simulink model "laba3"  (R2020b)
settings: Solver=VariableStepAuto  StartTime=0.0  StopTime=20  RelTol=1e-3
undefined symbols (not defined in the file): A, b, C, G, L, V, W
libraries: simulink x2
settings Model: Creator=Dimuss  LastModifiedBy=Dimuss
settings DebuggingCC: UnconnectedInputMsg=none  UnconnectedOutputMsg=none  UnconnectedLineMsg=none  SFMachineParentedDataDiag=error
settings ModelReferenceCC: EnableRefExpFcnMdlSchedulingChecks=off

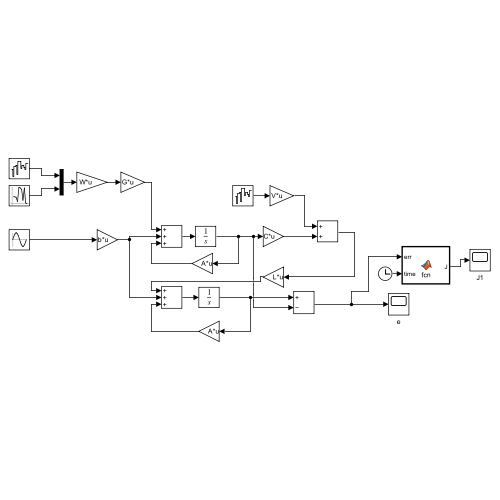
[thumbnail: Simulink's stored preview of the top-level diagram]
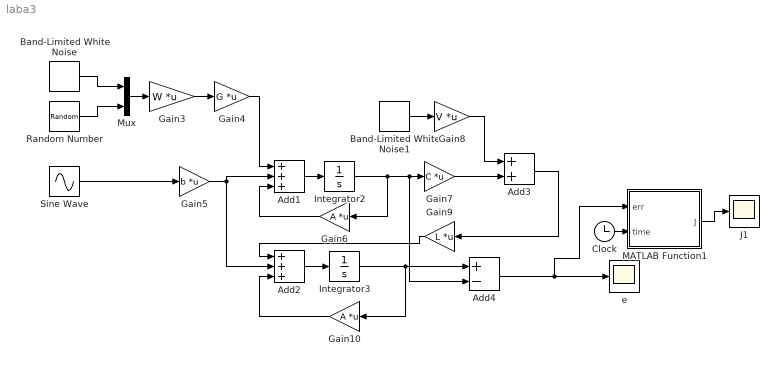
== system laba3 ==
  Add1 : Sum  Inputs=+++
  Add2 : Sum  Inputs=+++
  Add3 : Sum
  Add4 : Sum  Inputs=+-
  Band-Limited White Noise : simulink/Sources/Band-Limited White Noise  Cov=[0.1]  Ts=0.1  seed=[23341]
  Band-Limited White Noise1 : simulink/Sources/Band-Limited White Noise  Cov=[0.1]  Ts=0.1  seed=[23341]
  Clock : Clock
  Gain10 : Gain  Gain=A  Multiplication=Matrix(K*u)
  Gain3 : Gain  Gain=W  Multiplication=Matrix(K*u)
  Gain4 : Gain  Gain=G  Multiplication=Matrix(K*u)
  Gain5 : Gain  Gain=b  Multiplication=Matrix(K*u)
  Gain6 : Gain  Gain=A  Multiplication=Matrix(K*u)
  Gain7 : Gain  Gain=C  Multiplication=Matrix(K*u)
  Gain8 : Gain  Gain=V  Multiplication=Matrix(K*u)
  Gain9 : Gain  Gain=L  Multiplication=Matrix(K*u)
  Integrator2 : Integrator  InitialCondition=[1; 0]
  Integrator3 : Integrator  InitialCondition=[1; 0]
  J1 : Scope
  MATLAB Function1 : MATLAB Function  TreatAsAtomicUnit=on
  Mux : Mux  Inputs=2
  Random Number : RandomNumber  SampleTime=0.1
  Sine Wave : Sin  SampleTime=0
  e : Scope
  wires:
  Band-Limited White Noise/1 -> Mux/1
  Random Number/1 -> Mux/2
  Mux/1 -> Gain3/1
  Gain3/1 -> Gain4/1
  Gain4/1 -> Add1/1
  Gain5/1 -> Add2/2, Add1/2
  Sine Wave/1 -> Gain5/1
  Add1/1 -> Integrator2/1
  Integrator2/1 -> Add4/2, Gain7/1, Gain6/1
  Gain6/1 -> Add1/3
  Band-Limited White Noise1/1 -> Gain8/1
  Gain7/1 -> Add3/2
  Gain8/1 -> Add3/1
  Add3/1 -> Gain9/1
  Gain9/1 -> Add2/1
  Add2/1 -> Integrator3/1
  Gain10/1 -> Add2/3
  Integrator3/1 -> Add4/1, Gain10/1
  Add4/1 -> MATLAB Function1/1(err), e/1
  MATLAB Function1/1(J) -> J1/1
  Clock/1 -> MATLAB Function1/2(time)

== matlab function laba3/MATLAB Function1 ==
  data: J output; err input; time input
function J = fcn(err, time)
err = err'*err;
J = err/time;
